simulink model "with_demand_res_final_v5"  (R2024a)
settings: Solver=VariableStepAuto  StartTime=0.0  StopTime=24  RelTol=1e-3
InitFcn:
  | set_param(bdroot, 'StopTime', num2str(stop_time));
values from neighbouring files (symbols this model uses):
  fnom = 50    [initial_conditions.m]
  L_H_20kv = X_20kv_ohm/(2*pi*fnom)    (= 0.00126369024815)    [initial_conditions.m]
  L_H_400v = X_400v_ohm/(2*pi*fnom)    (= 0.00022600001919)    [initial_conditions.m]
  Pload_opt_nngwo_comb_cost = Pload_opt_nn    [gwo_nn_comb_cost.m]
  R_20kv = 0.576    [initial_conditions.m]
  R_400v = 0.410    (= 0.41)    [initial_conditions.m]
  Vph_ph_rms_nom_supply = 20e3    (= 20000)    [initial_conditions.m]
undefined symbols (not defined in the file or in its folder): D1, Delta
libraries: spsRMSLib x14, spsThreePhaseVIMeasurementLib x8, spsPowerPositiveSequenceLib x7, spsPLL3phLib x6, spsStairGeneratorLib x4, spsSeriesRLCBranchLib x3, spsThreePhasePISectionLineLib x2, spsThreePhaseTransformerTwoWindingsLib x2, spsThreePhaseSeriesRLCBranchLib x2, spsThreePhaseSeriesRLCLoadLib x2, slpidlib x2, spsabctodq0Lib x2
(part 1 of 2)
settings Model: Creator=arisi  LastModifiedBy=arisi
settings DataIOCC: ReturnWorkspaceOutputsName=with_demand_res

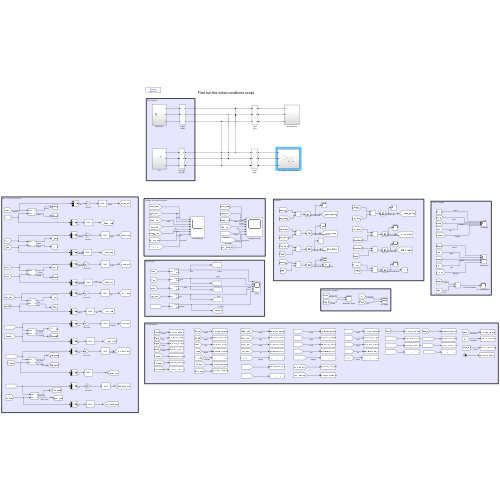
[thumbnail: Simulink's stored preview of the top-level diagram]
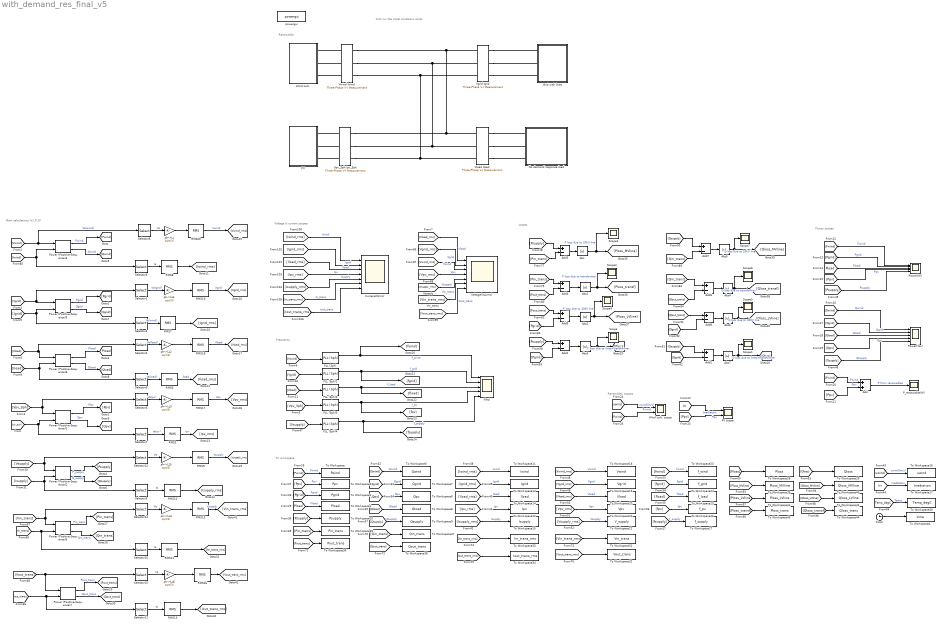
== system with_demand_res_final_v5 ==
  note: Voltage & current scopes
  note: First run the initial conditions script
  note: Losses
  note: Main calculations (V,I,P,Q)
  note: Frequency
  note: To workspace
  note: Renewable
  note: Renewbles' scopes
  note: Power scopes
  Abs{,1..7} (8 alike) : Abs  SaturateOnIntegerOverflow=off
  Add : Sum
  Add{1..8} (8 alike) : Sum  Inputs=+-
  Clock : Clock
  Currenet(Irms) : Scope  NumInputPorts=7
  Grid with lines : Subsystem
  No demand response load : Subsystem
  PLL (3ph){,1..4} (5 alike) : spsPLL3phLib/PLL (3ph)  Fmin=45  Par_Init=[0, 50]  ParK=[180, 3200, 1]  TcD=1e-4  MaxRateChangeFreq=12  FilterCutOffFreq=25  Ts=0  AGC=on
  PV : Subsystem
  PV scope : Scope  NumInputPorts=2
  P_renewable(W) : Scope
  Power (Positive-Sequence){1..7} (7 alike) : spsPowerPositiveSequenceLib/Power (Positive-Sequence)  Freq=50  Vinit=[0, 0]  Iinit=[0, 0]  Ts=0
      settings: LibrarySourceBlock=|
      | sps_lib/Sensors and Measurements/Power
      | (Positive-Sequence)
  Power(Var) : Scope  NumInputPorts=5
  Power(W) : Scope  NumInputPorts=5
  RMS{2,6..8,10..11,13} (7 alike) : spsRMSLib/RMS  TrueRMS=on  Freq=50  RMSInit=0  Ts=0
  RMS15 : spsRMSLib/RMS  TrueRMS=on  Freq=50  RMSInit=20e3  Ts=0
  RMS{16..20} (5 alike) : spsRMSLib/RMS  TrueRMS=on  Freq=50  RMSInit=400  Ts=0
  RMS9 : spsRMSLib/RMS  TrueRMS=on  Freq=50  RMSInit=20e3  Ts=0
  Scope{,1..7} (8 alike) : Scope
  Selector{1..12,14..15} (14 alike) : Selector  InputPortWidth=3  IndexOptions=Index vector (dialog)  Indices=1  OutputSizes=1
  To Workspace : ToWorkspace  VariableName=Pwind  SampleTime=-1
      settings: Save2DSignal=2-D array (concatenate along first dimension)
  To Workspace1 : ToWorkspace  VariableName=Pload  SampleTime=-1
      settings: Save2DSignal=2-D array (concatenate along first dimension)
  To Workspace10 : ToWorkspace  VariableName=Psupply  SampleTime=-1
      settings: Save2DSignal=2-D array (concatenate along first dimension)
  To Workspace11 : ToWorkspace  VariableName=Iwind  SampleTime=-1
      settings: Save2DSignal=2-D array (concatenate along first dimension)
  To Workspace12 : ToWorkspace  VariableName=Ipv  SampleTime=-1
      settings: Save2DSignal=2-D array (concatenate along first dimension)
  To Workspace13 : ToWorkspace  VariableName=Igrid  SampleTime=-1
      settings: Save2DSignal=2-D array (concatenate along first dimension)
  To Workspace14 : ToWorkspace  VariableName=Iload  SampleTime=-1
      settings: Save2DSignal=2-D array (concatenate along first dimension)
  To Workspace15 : ToWorkspace  VariableName=Isupply  SampleTime=-1
      settings: Save2DSignal=2-D array (concatenate along first dimension)
  To Workspace16 : ToWorkspace  VariableName=uwind  SampleTime=-1
      settings: Save2DSignal=2-D array (concatenate along first dimension)
  To Workspace17 : ToWorkspace  VariableName=Irradiation  SampleTime=-1
      settings: Save2DSignal=2-D array (concatenate along first dimension)
  To Workspace18 : ToWorkspace  VariableName=Vwind  SampleTime=-1
      settings: Save2DSignal=2-D array (concatenate along first dimension)
  To Workspace19 : ToWorkspace  VariableName=Vgrid  SampleTime=-1
      settings: Save2DSignal=2-D array (concatenate along first dimension)
  To Workspace2 : ToWorkspace  VariableName=Pgrid  SampleTime=-1
      settings: Save2DSignal=2-D array (concatenate along first dimension)
  To Workspace20 : ToWorkspace  VariableName=Vload  SampleTime=-1
      settings: Save2DSignal=2-D array (concatenate along first dimension)
  To Workspace21 : ToWorkspace  VariableName=Vpv  SampleTime=-1
      settings: Save2DSignal=2-D array (concatenate along first dimension)
  To Workspace22 : ToWorkspace  VariableName=V_supply  SampleTime=-1
      settings: Save2DSignal=2-D array (concatenate along first dimension)
  To Workspace23 : ToWorkspace  VariableName=f_wind  SampleTime=-1
      settings: Save2DSignal=2-D array (concatenate along first dimension)
  To Workspace24 : ToWorkspace  VariableName=f_grid  SampleTime=-1
      settings: Save2DSignal=2-D array (concatenate along first dimension)
  To Workspace25 : ToWorkspace  VariableName=f_load  SampleTime=-1
      settings: Save2DSignal=2-D array (concatenate along first dimension)
  To Workspace26 : ToWorkspace  VariableName=f_pv  SampleTime=-1
      settings: Save2DSignal=2-D array (concatenate along first dimension)
  To Workspace27 : ToWorkspace  VariableName=f_supply  SampleTime=-1
      settings: Save2DSignal=2-D array (concatenate along first dimension)
  To Workspace28 : ToWorkspace  VariableName=Ploss  SampleTime=-1
      settings: Save2DSignal=2-D array (concatenate along first dimension)
  To Workspace29 : ToWorkspace  VariableName=Qloss  SampleTime=-1
      settings: Save2DSignal=2-D array (concatenate along first dimension)
  To Workspace3 : ToWorkspace  VariableName=Ppv  SampleTime=-1
      settings: Save2DSignal=2-D array (concatenate along first dimension)
  To Workspace30 : ToWorkspace  VariableName=Temp_degC  SampleTime=-1
      settings: Save2DSignal=2-D array (concatenate along first dimension)
  To Workspace31 : ToWorkspace  VariableName=Vin_trans  SampleTime=-1
      settings: Save2DSignal=2-D array (concatenate along first dimension)
  To Workspace32 : ToWorkspace  VariableName=Vout_trans  SampleTime=-1
      settings: Save2DSignal=2-D array (concatenate along first dimension)
  To Workspace33 : ToWorkspace  VariableName=Iin_trans_rms  SampleTime=-1
      settings: Save2DSignal=2-D array (concatenate along first dimension)
  To Workspace34 : ToWorkspace  VariableName=Iout_trans_rms  SampleTime=-1
      settings: Save2DSignal=2-D array (concatenate along first dimension)
  To Workspace35 : ToWorkspace  VariableName=Pin_trans  SampleTime=-1
      settings: Save2DSignal=2-D array (concatenate along first dimension)
  To Workspace36 : ToWorkspace  VariableName=Pout_trans  SampleTime=-1
      settings: Save2DSignal=2-D array (concatenate along first dimension)
  To Workspace37 : ToWorkspace  VariableName=Qin_trans  SampleTime=-1
      settings: Save2DSignal=2-D array (concatenate along first dimension)
  To Workspace38 : ToWorkspace  VariableName=Qout_trans  SampleTime=-1
      settings: Save2DSignal=2-D array (concatenate along first dimension)
  To Workspace39 : ToWorkspace  VariableName=Ploss_MVline  SampleTime=-1
      settings: Save2DSignal=2-D array (concatenate along first dimension)
  To Workspace4 : ToWorkspace  VariableName=time  SampleTime=-1
      settings: Save2DSignal=2-D array (concatenate along first dimension)
  To Workspace40 : ToWorkspace  VariableName=Qloss_MVline  SampleTime=-1
      settings: Save2DSignal=2-D array (concatenate along first dimension)
  To Workspace41 : ToWorkspace  VariableName=Ploss_LVline  SampleTime=-1
      settings: Save2DSignal=2-D array (concatenate along first dimension)
  To Workspace42 : ToWorkspace  VariableName=Qloss_LVline  SampleTime=-1
      settings: Save2DSignal=2-D array (concatenate along first dimension)
  To Workspace43 : ToWorkspace  VariableName=Ploss_trans  SampleTime=-1
      settings: Save2DSignal=2-D array (concatenate along first dimension)
  To Workspace44 : ToWorkspace  VariableName=Qloss_trans  SampleTime=-1
      settings: Save2DSignal=2-D array (concatenate along first dimension)
  To Workspace5 : ToWorkspace  VariableName=Qwind  SampleTime=-1
      settings: Save2DSignal=2-D array (concatenate along first dimension)
  To Workspace6 : ToWorkspace  VariableName=Qpv  SampleTime=-1
      settings: Save2DSignal=2-D array (concatenate along first dimension)
  To Workspace7 : ToWorkspace  VariableName=Qgrid  SampleTime=-1
      settings: Save2DSignal=2-D array (concatenate along first dimension)
  To Workspace8 : ToWorkspace  VariableName=Qload  SampleTime=-1
      settings: Save2DSignal=2-D array (concatenate along first dimension)
  To Workspace9 : ToWorkspace  VariableName=Qsupply  SampleTime=-1
      settings: Save2DSignal=2-D array (concatenate along first dimension)
  Vgrid Igrid : spsThreePhaseVIMeasurementLib/Three-Phase V-I Measurement  VoltageMeasurement=phase-to-ground  SetLabelV=on  LabelV=Vgrid  Vpu=off  VpuLL=off  CurrentMeasurement=yes  SetLabelI=on  LabelI=Igrid  Ipu=off  Pbase=100e6  Vbase=500e3  OutputType=Complex  PhasorSimulation=off  PSBequivalent=0
  Vload Iload : spsThreePhaseVIMeasurementLib/Three-Phase V-I Measurement  VoltageMeasurement=phase-to-ground  SetLabelV=on  LabelV=Vload  Vpu=off  VpuLL=off  CurrentMeasurement=yes  SetLabelI=on  LabelI=Iload  Ipu=off  Pbase=100e6  Vbase=500e3  OutputType=Complex  PhasorSimulation=off  PSBequivalent=0
  Voltage(VLLrms) : Scope  NumInputPorts=7
  Vpv_3ph Ipv_3ph : spsThreePhaseVIMeasurementLib/Three-Phase V-I Measurement  VoltageMeasurement=phase-to-ground  SetLabelV=on  LabelV=Vpv_3ph  Vpu=off  VpuLL=off  CurrentMeasurement=yes  SetLabelI=on  LabelI=Ipv_3ph  Ipu=off  Pbase=100e6  Vbase=500e3  OutputType=Complex  PhasorSimulation=off  PSBequivalent=0
  Vwind Iwind : spsThreePhaseVIMeasurementLib/Three-Phase V-I Measurement  VoltageMeasurement=phase-to-ground  SetLabelV=on  LabelV=Vwind  Vpu=off  VpuLL=off  CurrentMeasurement=yes  SetLabelI=on  LabelI=Iwind  Ipu=off  Pbase=100e6  Vbase=500e3  OutputType=Complex  PhasorSimulation=off  PSBequivalent=0
  Wind turb. : Subsystem
  Wind turb. scope : Scope  NumInputPorts=2
  f(Hz) : Scope  NumInputPorts=5
  ph->LL{,1..6} (7 alike) : Gain  Gain=sqrt(3)
  powergui : spspowerguiLib/powergui  Priority=1  SimulationMode=Discrete  SampleTime=6.06e-6  frequency=60  Iterations=50  frequencyindice=50  Pbase=100e6  ErrMax=1e-4  UnitsV=kV  UnitsW=MW  buscounter=0  FunctionMessages=off  echomessages=off  EnableUseOfTLC=off  CurrentSourceSwitches=off  DisableSnubberDevices=off  DisableRonSwitches=off  DisableVfSwitches=off  DisplayEquations=off  AutomaticDiscreteSolvers=off  SolverType=Tustin  Interpol=off  ExternalGateDelay=off  methode=off  Ts=0  x0status=blocks  SPID=off  SwTol=0  HookPort=off  NonlinearTolerance=1e-4  nMaxIteration=15  ContinueOnMaxIteration=off  RestoreLinks=warning  ResistiveCurrentMeasurement=off  Frange=[0:2:500]  Ylog=off  Xlog=on  ShowGrid=off  save=off  variable=ZData  structure=VaIa_Grid  ZoomFFT=off  StartTime=1.4  cycles=3  DisplayStyle=1  fundamental=60  FreqAxis=on  MaxFrequency=5000  frequencyindicesteady=1  RmsSteady=1  display=off
  tag scope: Pload=global
  wires:
  Power (Positive-Sequence)5/2 -> [Qgrid]  "Qgrid"
  Selector6/1 -> ph->LL3/1  "Va(pv)"
  PLL (3ph)1/1 -> f(Hz)/2, [fgrid]  "f_grid"
  Power (Positive-Sequence)4/2 -> [Qwind]  "Qwind"
  [Irr] -> PV scope/1  "Irradiation"
  [Qpv] -> Power(Var)/4  "Qpv"
  [Ppv] -> PV scope/2  "Ppv"
  [Pwind] -> Wind turb. scope/2  "Pwind"
  Power (Positive-Sequence)1/2 -> [Qpv]  "Qpv"
  [Vpv_3ph] -> Power (Positive-Sequence)1/1, Selector6/1
  [Vload] -> Selector2/1, Power (Positive-Sequence)6/1
  [Ppv] -> Add/2  "Ppv"
  [uwind] -> Wind turb. scope/1  "uwind(m/s)"
  [Pload] -> Power(W)/3  "Pload"
  RMS7/1 -> [Igrid_rms]
  Selector2/1 -> ph->LL2/1  "Va(load)"
  ph->LL3/1 -> RMS17/1
  RMS6/1 -> [Iload_rms]  "Iload"
  Power (Positive-Sequence)6/2 -> [Qload]  "Qload"
  Power (Positive-Sequence)1/1 -> [Ppv]  "Plpv"
  Add/1 -> P_renewable(W)/1  "P from renewables"
  [Pwind] -> Add/1  "Pwind"
  [Qgrid] -> Power(Var)/2  "Qgrid"
  [Qwind] -> Power(Var)/1  "Qwind"
  [Qload] -> Power(Var)/3  "Qload"
  [Pgrid] -> Power(W)/2  "Pgrid"
  PLL (3ph)2/1 -> f(Hz)/3, [fload]  "f_load"
  Power (Positive-Sequence)5/1 -> [Pgrid]  "Pgrid"
  Selector1/1 -> ph->LL1/1  "Va(grid)"
  [Vgrid] -> Selector1/1, Power (Positive-Sequence)5/1
  RMS8/1 -> [Iwind_rms]
  [Vpv_3ph] -> PLL (3ph)3/1
  RMS2/1 -> [Ipv_rms]  "Ipv"
  [Pwind] -> Power(W)/1  "Pwind"
  [Vload] -> PLL (3ph)2/1
  Power (Positive-Sequence)4/1 -> [Pwind]  "Pwind"
  ph->LL1/1 -> RMS19/1
  PLL (3ph)3/1 -> [fpv], f(Hz)/4  "f_pv"
  ph->LL2/1 -> RMS18/1
  Selector5/1 -> RMS8/1  "Ia"
  [Ppv] -> Power(W)/4  "Ppv"
  Selector4/1 -> RMS7/1  "Ia(wind)"
  Selector3/1 -> RMS6/1  "Ia(load)"
  PLL (3ph)/1 -> f(Hz)/1, [fwind]  "f_wind"
  Selector7/1 -> RMS2/1  "Ia(pv)"
  [Vwind] -> Selector8/1, Power (Positive-Sequence)4/1  "Va(wind)"
  Power (Positive-Sequence)6/1 -> [Pload]  "Pload"
  [Vgrid] -> PLL (3ph)1/1
  [Vwind] -> PLL (3ph)/1
  [Pwind] -> To Workspace/1  "Pwind"
  [Ppv] -> To Workspace3/1  "Ppv"
  [Pgrid] -> To Workspace2/1  "Pgrid"
  [Pload] -> To Workspace1/1  "Pload"
  Clock/1 -> To Workspace4/1
  ph->LL5/1 -> RMS9/1
  Power (Positive-Sequence)2/1 -> [Psupply]  "P_supply"
  Selector12/1 -> ph->LL5/1  "Va"
  Power (Positive-Sequence)2/2 -> [Qsupply]  "Q_supply"
  [Vsupply] -> Selector12/1, Power (Positive-Sequence)2/1
  Selector9/1 -> RMS10/1  "Ia"
  RMS10/1 -> [Isupply_rms]
  [Qwind] -> To Workspace5/1  "Qwind"
  [Qgrid] -> To Workspace7/1  "Qgrid"
  [Qpv] -> To Workspace6/1  "Qpv"
  [Qload] -> To Workspace8/1  "Qload"
  [Qsupply] -> To Workspace9/1  "Qsupply"
  [Psupply] -> To Workspace10/1
  [Iwind_rms] -> To Workspace11/1  "Iwind"
  [Igrid_rms] -> To Workspace13/1  "Igrid"
  [Iload_rms] -> To Workspace14/1  "Iload"
  [Ipv_rms] -> To Workspace12/1  "Ipv"
  [Isupply_rms] -> To Workspace15/1  "Isupply"
  [uwind] -> To Workspace16/1  "uwind(m/s)"
  [Irr] -> To Workspace17/1  "Irradiation"
  [Psupply] -> Power(W)/5  "Psupply"
  [Qsupply] -> Power(Var)/5  "Qsupply"
  [Vsupply] -> PLL (3ph)4/1
  PLL (3ph)4/1 -> f(Hz)/5, [fsupply]  "f_supply"
  [Vwind_rms] -> To Workspace18/1  "Vwind"
  [Vgrid_rms] -> To Workspace19/1  "Vgrid"
  [Vload_rms] -> To Workspace20/1  "Vload"
  [Vpv_rms] -> To Workspace21/1  "Vpv"
  [Vsupply_rms] -> To Workspace22/1  "Vsupply"
  [fwind] -> To Workspace23/1  "fwind"
  [fgrid] -> To Workspace24/1  "fgrid"
  [fload] -> To Workspace25/1  "fload"
  [fpv] -> To Workspace26/1  "fpv"
  [fsupply] -> To Workspace27/1  "f_supply"
  [Psupply] -> Add1/1
  [Pgrid] -> Add1/2
  [Qsupply] -> Add2/1
  [Qgrid] -> Add2/2
  [Ploss] -> To Workspace28/1
  [Qloss] -> To Workspace29/1
  [Temp_degC] -> To Workspace30/1  "Temp"
  Selector11/1 -> RMS13/1  "Ia"
  Selector10/1 -> RMS11/1  "Ia"
  [Vout_trans] -> Power (Positive-Sequence)7/1, Selector15/1
  Power (Positive-Sequence)3/1 -> [Pin_trans]  "Pin_trans"
  Power (Positive-Sequence)3/2 -> [Qin_trans]  "Qin_trans"
  Power (Positive-Sequence)7/2 -> [Qout_trans]  "Qout_trans"
  Power (Positive-Sequence)7/1 -> [Pout_trans]  "Pout_trans"
  RMS11/1 -> [Iin_trans_rms]
  [Vin_trans_rms] -> To Workspace31/1
  RMS13/1 -> [Iout_trans_rms]
  [Iin_trans_rms] -> To Workspace33/1
  [Iout_trans_rms] -> To Workspace34/1
  [Vout_trans_rms] -> To Workspace32/1
  [Pin_trans] -> To Workspace35/1
  [Pout_trans] -> To Workspace36/1
  [Qin_trans] -> To Workspace37/1
  [Qout_trans] -> To Workspace38/1
  [Pin_trans] -> Add3/2
  [Psupply] -> Add3/1
  [Pin_trans] -> Add4/1
  [Pout_trans] -> Add4/2
  [Pout_trans] -> Add5/1
  [Pgrid] -> Add5/2
  [Qin_trans] -> Add6/1
  [Qout_trans] -> Add6/2
  [Qin_trans] -> Add7/2
  [Qsupply] -> Add7/1
  [Qgrid] -> Add8/2
  [Qout_trans] -> Add8/1
  [Ploss_MVline] -> To Workspace39/1
  [Qloss_MVline] -> To Workspace40/1
  [Qloss_LVline] -> To Workspace42/1
  [Ploss_LVline] -> To Workspace41/1
  [Qloss_transf] -> To Workspace44/1
  [Ploss_transf] -> To Workspace43/1
  [Iwind] -> Selector5/1, Power (Positive-Sequence)4/2
  [Igrid] -> Selector4/1, Power (Positive-Sequence)5/2
  [Iload] -> Selector3/1, Power (Positive-Sequence)6/2
  [Ipv_3ph] -> Selector7/1, Power (Positive-Sequence)1/2
  [Isupply] -> Selector9/1, Power (Positive-Sequence)2/2
  [Vin_trans] -> Selector14/1, Power (Positive-Sequence)3/1
  [Iin_trans] -> Selector10/1, Power (Positive-Sequence)3/2
  [Iout_trans] -> Selector11/1, Power (Positive-Sequence)7/2
  Selector14/1 -> ph->LL4/1  "Va"
  ph->LL4/1 -> RMS15/1
  Selector15/1 -> ph->LL6/1  "Va"
  ph->LL6/1 -> RMS16/1
  RMS19/1 -> [Vgrid_rms]  "Vgrid"
  RMS18/1 -> [Vload_rms]  "Vload"
  RMS17/1 -> [Vpv_rms]  "Vpv"
  RMS9/1 -> [Vsupply_rms]  "Vsupply"
  RMS15/1 -> [Vin_trans_rms]  "Vsupply"
  RMS16/1 -> [Vout_trans_rms]
  [Vload_rms] -> Voltage(VLLrms)/1  "Vload"
  [Vgrid_rms] -> Voltage(VLLrms)/2  "Vgrid"
  [Vwind_rms] -> Voltage(VLLrms)/3  "Vwind"
  [Vpv_rms] -> Voltage(VLLrms)/4  "Vpv"
  [Vsupply_rms] -> Voltage(VLLrms)/5  "Vsupply"
  [Vin_trans_rms] -> Voltage(VLLrms)/6  "Vin_trans"
  [Vout_trans_rms] -> Voltage(VLLrms)/7  "Vout_trans"
  [Iwind_rms] -> Currenet(Irms)/1  "Iwind"
  [Igrid_rms] -> Currenet(Irms)/2  "Igird"
  [Iload_rms] -> Currenet(Irms)/3  "Iload"
  [Ipv_rms] -> Currenet(Irms)/4  "Ipv"
  [Isupply_rms] -> Currenet(Irms)/5  "Isupply"
  [Iin_trans_rms] -> Currenet(Irms)/6  "In_trans"
  [Iout_trans_rms] -> Currenet(Irms)/7  "Iout_trans"
  Add3/1 -> Abs/1
  Abs/1 -> Scope2/1, [Ploss_MVline]  "P loss due to 20kV line"
  Add4/1 -> Abs1/1
  Abs1/1 -> Scope3/1, [Ploss_transf]  "P loss due to transformer"
  Add5/1 -> Abs2/1
  Abs2/1 -> Scope4/1, [Ploss_LVline]  "P loss due to 400V line"
  Add1/1 -> Abs3/1
  Abs3/1 -> Scope/1, [Ploss]  "P loss due to lines+transformer"
  Add2/1 -> Abs7/1
  Abs7/1 -> [Qloss], Scope1/1  "Q loss due to lines+transformer"
  Add8/1 -> Abs6/1
  Abs6/1 -> [Qloss_LVline], Scope5/1  "Q loss due to 400V line"
  Add6/1 -> Abs4/1
  Abs4/1 -> [Qloss_transf], Scope6/1  "Q loss due to transformer"
  Add7/1 -> Abs5/1
  Abs5/1 -> [Qloss_MVline], Scope7/1  "Q loss due to 20kV line"
  ph->LL/1 -> RMS20/1
  Selector8/1 -> ph->LL/1  "Va"
  RMS20/1 -> [Vwind_rms]  "Vwind"
  connections:
  Vload Iload/LConn2 -- Vpv_3ph Ipv_3ph/RConn2 -- Vwind Iwind/RConn2 -- Vgrid Igrid/RConn2
  Vload Iload/LConn3 -- Vpv_3ph Ipv_3ph/RConn3 -- Vwind Iwind/RConn3 -- Vgrid Igrid/RConn3
  Vload Iload/LConn1 -- Vwind Iwind/RConn1 -- Vgrid Igrid/RConn1 -- Vpv_3ph Ipv_3ph/RConn1
  Vload Iload/RConn1 -- No demand response load/LConn1
  Vload Iload/RConn2 -- No demand response load/LConn2
  Vload Iload/RConn3 -- No demand response load/LConn3
  Vwind Iwind/LConn2 -- Wind turb./LConn2
  Vpv_3ph Ipv_3ph/LConn3 -- PV/RConn3
  Vwind Iwind/LConn3 -- Wind turb./LConn3
  Vwind Iwind/LConn1 -- Wind turb./LConn1
  Vpv_3ph Ipv_3ph/LConn2 -- PV/RConn2
  Vpv_3ph Ipv_3ph/LConn1 -- PV/RConn1
  Vgrid Igrid/LConn3 -- Grid with lines/RConn3
  Vgrid Igrid/LConn1 -- Grid with lines/RConn1
  Vgrid Igrid/LConn2 -- Grid with lines/RConn2

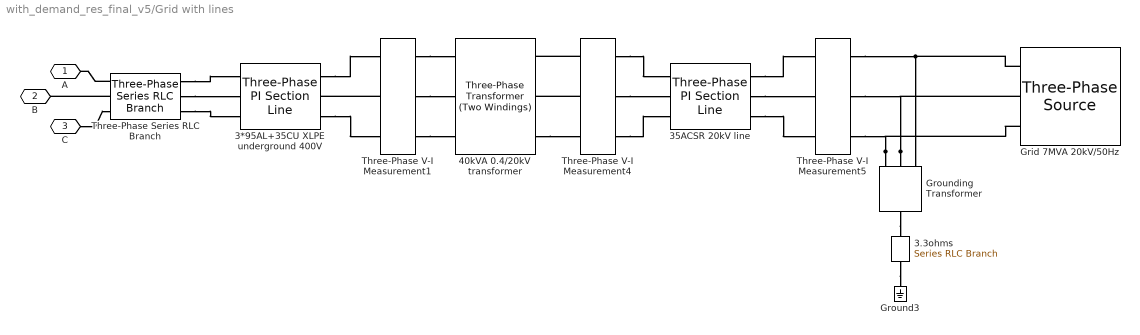
== system with_demand_res_final_v5/Grid with lines ==
  3*95AL+35CU XLPE underground 400V : spsThreePhasePISectionLineLib/Three-Phase PI Section Line  LConnTagsString=a|b|c  RConnTagsString=A|B|C  Length=km_400v  Frequency=fnom  Resistances=[ R_400v 0.724]  Inductances="[ L_H_400v  1.595/(2*pi*50)]"  Capacitances=[60e-9 7.751e-9]
  "3.3ohms " : spsSeriesRLCBranchLib/Series RLC Branch  LConnTagsString=__new0  RConnTagsString=__new0  BranchType=R  Resistance=3.3  Inductance=[]  SetiL0=off  InitialCurrent=0  Capacitance=[]  Setx0=off  InitialVoltage=0  Measurements=None
  35ACSR 20kV line : spsThreePhasePISectionLineLib/Three-Phase PI Section Line  LConnTagsString=a|b|c  RConnTagsString=A|B|C  Length=km_20kv  Frequency=fnom  Resistances=[ R_20kv 0.724]  Inductances="[ L_H_20kv  1.595/(2*pi*50)]"  Capacitances=[50e-9 7.751e-9]
  40kVA 0.4/20kV transformer : spsThreePhaseTransformerTwoWindingsLib/Three-Phase Transformer (Two Windings)  Winding1Connection=Yg  Winding2Connection=Delta (D1)  CoreType=Three single-phase transformers  SetSaturation=off  Hysteresis=off  DataFile='hysteresis'  SetInitialFlux=off  Measurements=None  UNITS=pu  NominalPower=nominal_trans_param  Winding1=winding_1_param  Winding2=winding_2_param  Rm=Lm_pu  Lm=Rm_pu  L0=0.5  Saturation=[ 0,0 ; 0.0024,1.2 ; 1.0,1.52 ]  InitialFluxes=[ 0.8 , -0.8 , 0.7 ]  BreakLoop=off  DiscreteSolver=Trapezoidal iterative  DataType=off  TransfoNumber=1
  "Grid 7MVA 20kV/50Hz " : spsThreePhaseSourceLib/Three-Phase Source  InternalConnection=Yg  VoltagePhases=off  Voltage=Vph_ph_rms_nom_supply  PhaseAngle=0  Voltage_phases=[25e3 25e3 25e3]/sqrt(3)  PhaseAngles_phases=[0 -120 +120]  Frequency=fnom  NonIdealSource=on  SpecifyImpedance=on  Resistance=0.8929  Inductance=16.58e-3  ShortCircuitLevel=Ssupply  BaseVoltage=Vph_ph_rms_nom_supply  XRratio=XRratio  BusType=swing  Pref=0  Qref=0  Prefabc=[10e3, 10e3, 10e3]  Qrefabc=[0, 0, 0]  Qmin=-inf  Qmax=inf
  Ground3 : spsGroundLib/Ground  LConnTagsString=a
  "Grounding Transformer " : spsGroundingTransformerLib/Grounding Transformer   UNITS=pu  NominalPower="[100e6   50]"  NominalVoltage=20e3  ZeroSequenceImpedance_pu=[0.025 0.75]  MagnetizationBranch_pu=[500 500]  ZeroSequenceImpedance_SI=[0.052083 589.05]  MagnetizationBranch_SI=[1041.7 3.927e+005]  Measurements=None
      settings: LibrarySourceBlock=|
      | sps_lib/Power Grid Elements/Grounding
      | Transformer
  Three-Phase Series RLC Branch : spsThreePhaseSeriesRLCBranchLib/Three-Phase Series RLC Branch  LConnTagsString=A|B|C  RConnTagsString=A|B|C  BranchType=R  Resistance=1e-3  Inductance=1e-3  Capacitance=1e-6  Measurements=None
  Three-Phase V-I Measurement1 : spsThreePhaseVIMeasurementLib/Three-Phase V-I Measurement  VoltageMeasurement=phase-to-ground  SetLabelV=on  LabelV=Vout_trans  Vpu=off  VpuLL=off  CurrentMeasurement=yes  SetLabelI=on  LabelI=Iout_trans  Ipu=off  Pbase=100e6  Vbase=500e3  OutputType=Complex  PhasorSimulation=off  PSBequivalent=0
  Three-Phase V-I Measurement4 : spsThreePhaseVIMeasurementLib/Three-Phase V-I Measurement  VoltageMeasurement=phase-to-ground  SetLabelV=on  LabelV=Vin_trans  Vpu=off  VpuLL=off  CurrentMeasurement=yes  SetLabelI=on  LabelI=Iin_trans  Ipu=off  Pbase=100e6  Vbase=500e3  OutputType=Complex  PhasorSimulation=off  PSBequivalent=0
  Three-Phase V-I Measurement5 : spsThreePhaseVIMeasurementLib/Three-Phase V-I Measurement  VoltageMeasurement=phase-to-ground  SetLabelV=on  LabelV=Vsupply  Vpu=off  VpuLL=off  CurrentMeasurement=yes  SetLabelI=on  LabelI=Isupply  Ipu=off  Pbase=100e6  Vbase=500e3  OutputType=Complex  PhasorSimulation=off  PSBequivalent=0
  A : PMIOPort  Side=Right
  B : PMIOPort  Port=2  Side=Right
  C : PMIOPort  Port=3  Side=Right
  connections:
  Three-Phase Series RLC Branch/RConn1 -- A/RConn1
  Three-Phase Series RLC Branch/LConn1 -- 3*95AL+35CU XLPE underground 400V/RConn1
  3*95AL+35CU XLPE underground 400V/LConn1 -- Three-Phase V-I Measurement1/RConn1
  "Grounding Transformer "/LConn2 -- "Grid 7MVA 20kV/50Hz "/RConn2 -- Three-Phase V-I Measurement5/LConn2
  "Grid 7MVA 20kV/50Hz "/RConn1 -- "Grounding Transformer "/LConn1 -- Three-Phase V-I Measurement5/LConn1
  Three-Phase V-I Measurement1/RConn2 -- 3*95AL+35CU XLPE underground 400V/LConn2
  Three-Phase V-I Measurement4/RConn1 -- 40kVA 0.4/20kV transformer/LConn1
  "Grounding Transformer "/RConn1 -- "3.3ohms "/LConn1
  35ACSR 20kV line/LConn3 -- Three-Phase V-I Measurement5/RConn3
  Three-Phase V-I Measurement1/LConn2 -- 40kVA 0.4/20kV transformer/RConn2
  Three-Phase V-I Measurement1/LConn1 -- 40kVA 0.4/20kV transformer/RConn1
  Three-Phase Series RLC Branch/LConn2 -- 3*95AL+35CU XLPE underground 400V/RConn2
  Three-Phase V-I Measurement4/LConn1 -- 35ACSR 20kV line/RConn1
  Three-Phase Series RLC Branch/LConn3 -- 3*95AL+35CU XLPE underground 400V/RConn3
  "Grounding Transformer "/LConn3 -- "Grid 7MVA 20kV/50Hz "/RConn3 -- Three-Phase V-I Measurement5/LConn3
  35ACSR 20kV line/LConn2 -- Three-Phase V-I Measurement5/RConn2
  35ACSR 20kV line/LConn1 -- Three-Phase V-I Measurement5/RConn1
  "3.3ohms "/RConn1 -- Ground3/LConn1
  Three-Phase V-I Measurement4/RConn2 -- 40kVA 0.4/20kV transformer/LConn2
  Three-Phase V-I Measurement4/LConn3 -- 35ACSR 20kV line/RConn3
  Three-Phase V-I Measurement4/LConn2 -- 35ACSR 20kV line/RConn2
  40kVA 0.4/20kV transformer/LConn3 -- Three-Phase V-I Measurement4/RConn3
  Three-Phase V-I Measurement1/LConn3 -- 40kVA 0.4/20kV transformer/RConn3
  Three-Phase Series RLC Branch/RConn2 -- B/RConn1
  3*95AL+35CU XLPE underground 400V/LConn3 -- Three-Phase V-I Measurement1/RConn3
  C/RConn1 -- Three-Phase Series RLC Branch/RConn3

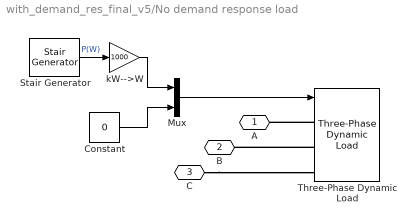
== system with_demand_res_final_v5/No demand response load ==
  Constant : Constant  Value=0
  Mux : Mux  Inputs=2
  Stair Generator : spsStairGeneratorLib/Stair Generator  t=no_drload_time  e=(Pload_opt_nngwo_comb_cost)'  Ts=0
  Three-Phase Dynamic Load : spsThreePhaseDynamicLoadLib/Three-Phase Dynamic Load  NominalVoltage=[ 400 50 ]  ActiveReactivePowers=[6e3 0]  PositiveSequence=[0.994 -11.8]  ExternalControl=on  NpNq=[1.3 2]  TimeConstants="[0  0  0  0]"  MinimumVoltage=0.7  Tfilter=1e-4  LoadFlowParameters=[4,0,0,0,0]
      settings: LibrarySourceBlock=|
      | sps_lib/Passives/Three-Phase
      | Dynamic Load
  kW-->W : Gain  Gain=1000
  A : PMIOPort  Side=Left
  B : PMIOPort  Port=2  Side=Left
  C : PMIOPort  Port=3  Side=Left
  wires:
  Mux/1 -> Three-Phase Dynamic Load/1
  Stair Generator/1 -> kW-->W/1  "P(W)"
  Constant/1 -> Mux/2
  kW-->W/1 -> Mux/1
  connections:
  C/RConn1 -- Three-Phase Dynamic Load/LConn3
  Three-Phase Dynamic Load/LConn1 -- A/RConn1
  Three-Phase Dynamic Load/LConn2 -- B/RConn1

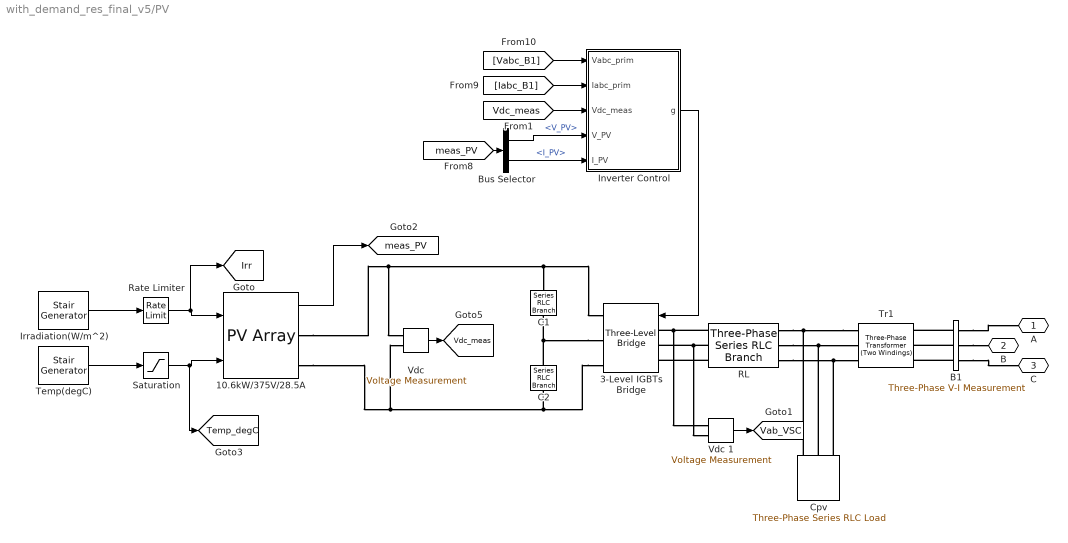
== system with_demand_res_final_v5/PV ==
  10.6kW/375V/28.5A : spsPVArrayLib/PV Array  Npar=4  Nser=13  PlotType=array @ 25 deg.C & specified irradiances  S_vec="[ 1000  500  100 ]"  Temp_C_vec="[ 45 25  ]"  ModuleName=Solartech Power SPM205P  PlotWhenSelected=off  Pm=205.056  Ncell=60  Voc=37.1  Isc=8.07  Vm=28.8  Im=7.12  beta_Voc_pc=-0.36403  alpha_Isc_pc=0.051128  beta_Voc=-0.13506  alpha_Isc=0.004126  IL=8.1521  I0=3.0369e-10  nI=1.006  Rsh=52.6281  Rs=0.53549  RobustModel=off  RobustCellTemperature=313.3991  BAL=on  Tc=1e-6  Tfilter=5e-5
  3-Level IGBTs Bridge : spsThreeLevelBridgeLib/Three-Level Bridge  Arms=3  SnubberResistance=1e6  SbubberCapacitance=inf  Device=IGBT / Diodes  Ron=1e-3  ForwardVoltages="[  0  0 ]"  Measurements=None
      settings: AttributesFormatString=\n  LibrarySourceBlock=sps_lib/Power Electronics/Three-Level Bridge
  B1 : spsThreePhaseVIMeasurementLib/Three-Phase V-I Measurement  VoltageMeasurement=phase-to-ground  SetLabelV=on  LabelV=Vabc_B1  Vpu=off  VpuLL=off  CurrentMeasurement=yes  SetLabelI=on  LabelI=Iabc_B1  Ipu=off  Pbase=100e6  Vbase=500e3  OutputType=Magnitude  PhasorSimulation=off  PSBequivalent=0
  Bus Selector : BusSelector  OutputSignals=V_PV,I_PV
  C1 : spsSeriesRLCBranchLib/Series RLC Branch  LConnTagsString=__new0  RConnTagsString=__new0  BranchType=C  Resistance=1.0  Inductance=1.0  SetiL0=off  InitialCurrent=0  Capacitance=0.00452266  Setx0=on  InitialVoltage=375/2  Measurements=None
  C2 : spsSeriesRLCBranchLib/Series RLC Branch  LConnTagsString=__new0  RConnTagsString=__new0  BranchType=C  Resistance=1.0  Inductance=1.0  SetiL0=off  InitialCurrent=0  Capacitance=0.00452266  Setx0=on  InitialVoltage=375/2  Measurements=None
  Cpv : spsThreePhaseSeriesRLCLoadLib/Three-Phase Series RLC Load  LConnTagsString=A|B|C  Configuration=Delta  NominalVoltage=195.1937  Vabc=[1e3 1e3 1e3]  Vabcp=[1e3 1e3 1e3]  NominalFrequency=50  UnbalancedPower=off  ActivePower=21.2  InductivePower=0  CapacitivePower=1060  Pabc=[10e3 9e3 11e3]  QLabc=[100 90 110]  QCabc=[100 90 110]  Pabcp=[10e3 9e3 11e3]  QLabcp=[100 90 110]  QCabcp=[100 90 110]  Measurements=None  LoadType=constant Z
  Inverter Control : Subsystem  mask(Inverter Control){Pnom=10600, Fnom=50, Vnom_prim=400, Vnom_sec=195.1937, Vnom_dc=375, Increment_MPPT=0.01, Limits_MPPT=[ 457 280 ], Vdc_ref_Init=375, Kp_VDCreg=2, Ki_VDCreg=400, Kp_Ireg=0.3, Ki_Ireg=20, RLff=[ 0.0039 0.21 ], Fc=1650, Ts_Control=6.06e-5, Ts_PWMgenerator=6.06e-6}
      mask prompts: Pnom "Power (VA)"; Fnom "Frequency (Hz)"; Vnom_prim "Primary voltage (Vrms LL)"; Vnom_sec "Secondary voltage (Vrms LL)"; Vnom_dc "DC voltage (V)"; Increment_MPPT "Output increment (V)"; Limits_MPPT "Output limits [ Upper  Lower ]"; Vdc_ref_Init "Output initial value (V)"; Kp_VDCreg "Proportional gain"; Ki_VDCreg "Integral gain"; Kp_Ireg "Proportional gain"; Ki_Ireg "Integral gain"; RLff "Feedforward Values [Rff Lff]"; Fc "Carrier frequency (Hz)"; Ts_Control "Control systems"; Ts_PWMgenerator "PWM generator"
      mask help:
      | The main components of the Inverter Control are:
      | 1. PLL & Measurements
      | 2. Maximum Power Point Tracker System (MPPT) using a Perturb & Observe algorithm
      | 3. DC Voltage Regulator
      | 4. Current Regulator
      | 5. PWM Modulator
      mask DialogControl Container4 Prompt: Nominal Values:
      mask DialogControl Container3 Prompt: MPPT Controller:
      mask DialogControl Container8 Prompt: Dc Voltage Regulator:
      mask DialogControl Container6 Prompt: Current Regulator:
      mask DialogControl Container9 Prompt: PWM Modulator:
      mask DialogControl SampleTimes Prompt: Sample Times:
  Irradiation(W/m^2) : spsStairGeneratorLib/Stair Generator  t=irradiation_time  e=irradiation_amplitude  Ts=0
  RL : spsThreePhaseSeriesRLCBranchLib/Three-Phase Series RLC Branch  LConnTagsString=A|B|C  RConnTagsString=A|B|C  BranchType=RL  Resistance=0.0053916  Inductance=0.001716197  Capacitance=inf  Measurements=None
  Rate Limiter : RateLimiter  RisingSlewLimit=6000  FallingSlewLimit=-6000  SampleTimeMode=inherited  InitialCondition=1000
  Saturation : Saturate  UpperLimit=55  LowerLimit=5
  Temp(degC) : spsStairGeneratorLib/Stair Generator  t=temperature_time  e=temperature_amplitude  Ts=0
  Tr1 : spsThreePhaseTransformerTwoWindingsLib/Three-Phase Transformer (Two Windings)  Winding1Connection=Yg  Winding2Connection=Delta (D1)  CoreType=Three single-phase transformers  SetSaturation=off  Hysteresis=off  DataFile='hysteresis'  SetInitialFlux=off  Measurements=None  UNITS=pu  NominalPower=[ 10600 50 ]  Winding1=[ 400 0.0012 0.03 ]  Winding2=[ 195.1937 0.0012 0.03 ]  Rm=200  Lm=200  L0=0.5  Saturation=[ 0,0 ; 0.0024,1.2 ; 1.0,1.52 ]  InitialFluxes=[ 0.8 , -0.8 , 0.7 ]  BreakLoop=off  DiscreteSolver=Trapezoidal iterative  DataType=off  TransfoNumber=0
  "Vdc " : spsVoltageMeasurementLib/Voltage Measurement  Tag=PoWeRsYsTeMmEaSuReMeNt  PhasorSimulation=off  OutputType=Magnitude  PSBequivalent=0
  Vdc 1 : spsVoltageMeasurementLib/Voltage Measurement  Tag=PoWeRsYsTeMmEaSuReMeNt  PhasorSimulation=off  OutputType=Magnitude  PSBequivalent=0
  A : PMIOPort  Side=Right
  B : PMIOPort  Port=2  Side=Right
  C : PMIOPort  Port=3  Side=Right
  tag scope: Irr=global, Temp_degC=global, Vab_VSC=global, Vdc_meas=global, meas_PV=global
  wires:
  Bus Selector/2 -> Inverter Control/5(I_PV)  "<I_PV>"
  Inverter Control/1(g) -> 3-Level IGBTs Bridge/1
  Rate Limiter/1 -> [Irr], 10.6kW/375V/28.5A/1
  Irradiation(W/m^2)/1 -> Rate Limiter/1
  [meas_PV] -> Bus Selector/1
  [Iabc_B1] -> Inverter Control/2(Iabc_prim)
  "Vdc "/1 -> [Vdc_meas]
  Vdc 1/1 -> [Vab_VSC]
  10.6kW/375V/28.5A/1 -> [meas_PV]
  [Vabc_B1] -> Inverter Control/1(Vabc_prim)
  [Vdc_meas] -> Inverter Control/3(Vdc_meas)
  Saturation/1 -> [Temp_degC], 10.6kW/375V/28.5A/2
  Temp(degC)/1 -> Saturation/1
  Bus Selector/1 -> Inverter Control/4(V_PV)  "<V_PV>"
  connections:
  3-Level IGBTs Bridge/RConn2 -- C1/RConn1 -- C2/LConn1
  "Vdc "/LConn1 -- 10.6kW/375V/28.5A/RConn1 -- 3-Level IGBTs Bridge/RConn1 -- C1/LConn1
  Cpv/LConn3 -- Tr1/RConn3 -- RL/RConn3
  Tr1/RConn1 -- Cpv/LConn1 -- RL/RConn1
  3-Level IGBTs Bridge/RConn3 -- 10.6kW/375V/28.5A/RConn2 -- "Vdc "/LConn2 -- C2/RConn1
  3-Level IGBTs Bridge/LConn2 -- RL/LConn2 -- Vdc 1/LConn2
  RL/RConn2 -- Tr1/RConn2 -- Cpv/LConn2
  3-Level IGBTs Bridge/LConn1 -- Vdc 1/LConn1 -- RL/LConn1
  B1/RConn1 -- A/RConn1
  B1/LConn2 -- Tr1/LConn2
  B1/LConn1 -- Tr1/LConn1
  RL/LConn3 -- 3-Level IGBTs Bridge/LConn3
  B1/LConn3 -- Tr1/LConn3
  B1/RConn2 -- B/RConn1
  B1/RConn3 -- C/RConn1

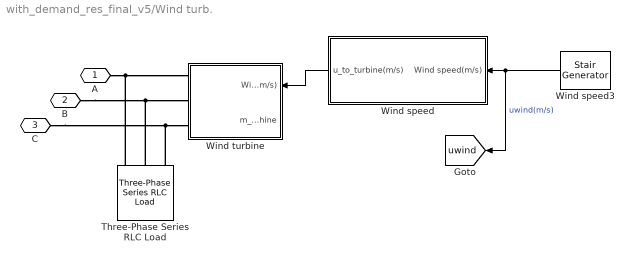
== system with_demand_res_final_v5/Wind turb. ==
  Three-Phase Series RLC Load : spsThreePhaseSeriesRLCLoadLib/Three-Phase Series RLC Load  LConnTagsString=A|B|C  Configuration=Y (grounded)  NominalVoltage=400  Vabc=[1e3 1e3 1e3]  Vabcp=[1e3 1e3 1e3]  NominalFrequency=50  UnbalancedPower=off  ActivePower=1e-6  InductivePower=0  CapacitivePower=18.6e3  Pabc=[10e3 9e3 11e3]  QLabc=[100 90 110]  QCabc=[100 90 110]  Pabcp=[10e3 9e3 11e3]  QLabcp=[100 90 110]  QCabcp=[100 90 110]  Measurements=None  LoadType=constant Z
  Wind speed : Subsystem
  Wind speed3 : spsStairGeneratorLib/Stair Generator  t=uwind_time  e=uwind_amplitude  Ts=0
  Wind turbine : Subsystem
      settings: PortSchema="{\"entries\":[{\"content\":{\"sides\":[{\"content\":{\"connectorIds\":[\"LConn1\",\"LConn2\",\"LConn3\"]},\"type\":\"ConnectorPlacement.EquallySpacedRectSide\",\"uuid\":\"08b69726-1df5-4ca6-8c10-95a87e57958a\"},{\"content\":{\"connectorIds\":[\"In1\",\"Out1\"],\"side\":\"RIGHT\"},\"type\":\"ConnectorPlacement.EquallySpacedRectSide\",\"uuid\":\"4b04fe79-4781-4367-afff-b10c5d568099\"},{\"content\":{\"side\":\"TOP\"},\"type\":\"ConnectorPlacement.EquallySpacedRectSide\",\"uuid\":\"2a53e08c-afc6-4d8a-b9a1-c6221c3edf36\"}]},\"type\":\"ConnectorPlacement.EquallySpacedConnector\",\"uuid\":\"1c063288-1d34-4ac9-8903-84a9f43e3a12\"}],\"packageUris\":[\"http://schema.mathworks.com/mf0/Connector/R2020b\"],\"version\":\"1.0\"}"
  A : PMIOPort  Side=Left
  B : PMIOPort  Port=2  Side=Left
  C : PMIOPort  Port=3  Side=Left
  tag scope: uwind=global
  wires:
  Wind speed/1(u_to_turbine(m/s)) -> Wind turbine/1("Wind (m/s) ")
  Wind speed3/1 -> [uwind], Wind speed/1(Wind speed(m/s))  "uwind(m/s)"
  connections:
  Three-Phase Series RLC Load/LConn2 -- B/RConn1 -- Wind turbine/LConn2
  Three-Phase Series RLC Load/LConn3 -- C/RConn1 -- Wind turbine/LConn3
  Three-Phase Series RLC Load/LConn1 -- A/RConn1 -- Wind turbine/LConn1

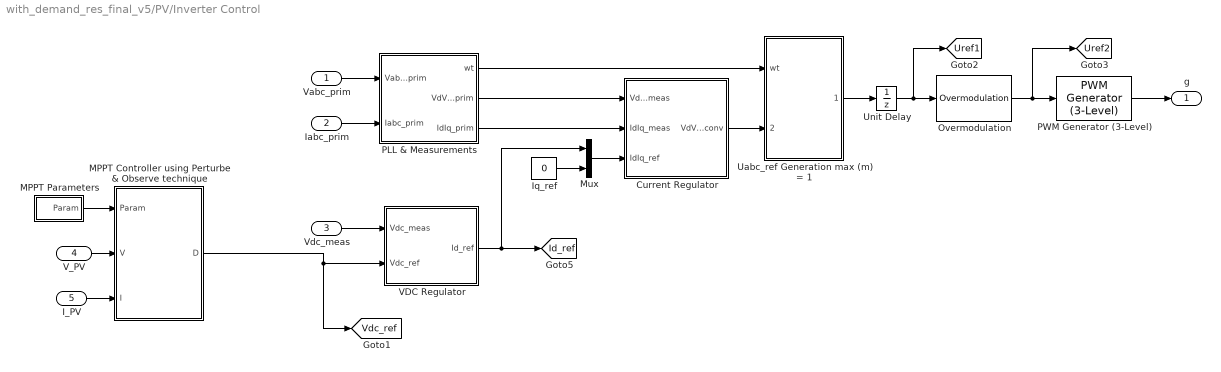
== system with_demand_res_final_v5/PV/Inverter Control ==
  Vabc_prim : Inport  PortDimensions=3
  Iabc_prim : Inport  Port=2  PortDimensions=3
  Vdc_meas : Inport  Port=3  PortDimensions=1
  V_PV : Inport  Port=4  PortDimensions=1
  I_PV : Inport  Port=5  PortDimensions=1
  Current Regulator : Subsystem
  Iq_ref : Constant  Value=0
  MPPT Parameters : Subsystem
  "MPPT Controller using Perturbe & Observe technique " : MATLAB Function  TreatAsAtomicUnit=on
  Mux : Mux  Inputs=2
  Overmodulation : spsOvermodulationLib/Overmodulation  OverModType=Flat top
      settings: LibrarySourceBlock=sps_lib/Power Electronics/Power Electronics Control/Overmodulation
  PLL & Measurements : Subsystem
  PWM Generator (3-Level) : spsPWMGenerator3LevelLib/PWM Generator (3-Level)  ModulatorType=Three-phase bridge (12 pulses)  ModulatorMode=Unsynchronized  nF=27  Fc=1650  ModulatingSignals=off  m=0.8  Freq=60  Phase=0  Ts=6.06e-6
      settings: LibrarySourceBlock=|
      | sps_lib/Power Electronics/Power Electronics Control/PWM Generator
      | (3-Level)
  Uabc_ref Generation max (m) = 1 : Subsystem
  Unit Delay : UnitDelay  SampleTime=6.06e-5  HasFrameUpgradeWarning=on
  VDC Regulator : Subsystem
  g : Outport  VectorParamsAs1DForOutWhenUnconnected=off
  tag scope: Id_ref=global, Uref1=global, Uref2=global, Vdc_ref=global
  wires:
  PLL & Measurements/1(wt) -> Uabc_ref Generation max (m) = 1/1(wt)
  Current Regulator/1(VdVq_conv) -> Uabc_ref Generation max (m) = 1/2(VdVq_conv)
  Iq_ref/1 -> Mux/2
  Mux/1 -> Current Regulator/3(IdIq_ref)
  PLL & Measurements/3(IdIq_prim) -> Current Regulator/2(IdIq_meas)
  PLL & Measurements/2(VdVq_prim) -> Current Regulator/1(VdVq_meas)
  Vabc_prim/1 -> PLL & Measurements/1(Vabc_prim)
  Iabc_prim/1 -> PLL & Measurements/2(Iabc_prim)
  PWM Generator (3-Level)/1 -> g/1
  Vdc_meas/1 -> VDC Regulator/1(Vdc_meas)
  VDC Regulator/1(Id_ref) -> [Id_ref], Mux/1
  V_PV/1 -> "MPPT Controller using Perturbe & Observe technique "/2(V)
  I_PV/1 -> "MPPT Controller using Perturbe & Observe technique "/3(I)
  MPPT Parameters/1(Param) -> "MPPT Controller using Perturbe & Observe technique "/1(Param)
  Overmodulation/1 -> [Uref2], PWM Generator (3-Level)/1
  Unit Delay/1 -> [Uref1], Overmodulation/1
  "MPPT Controller using Perturbe & Observe technique "/1(D) -> [Vdc_ref], VDC Regulator/2(Vdc_ref)
  Uabc_ref Generation max (m) = 1/1(Uabc_ref) -> Unit Delay/1

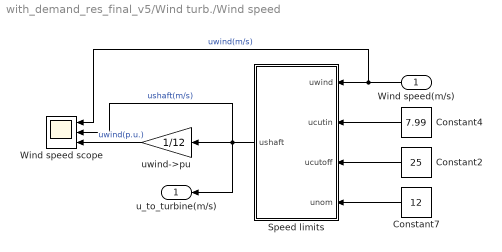
== system with_demand_res_final_v5/Wind turb./Wind speed ==
  Wind speed(m/s) : Inport
  Constant2 : Constant  Value=25
  Constant4 : Constant  Value=7.99
  Constant7 : Constant  Value=12
  Speed limits : MATLAB Function  TreatAsAtomicUnit=on
  Wind speed scope : Scope  NumInputPorts=3
  uwind->pu : Gain  Gain=1/12
  u_to_turbine(m/s) : Outport
  wires:
  Speed limits/1(ushaft) -> u_to_turbine(m/s)/1, uwind->pu/1, Wind speed scope/2  "ushaft(m/s)"
  Wind speed(m/s)/1 -> Wind speed scope/1, Speed limits/1(uwind)  "uwind(m/s)"
  Constant4/1 -> Speed limits/2(ucutin)
  uwind->pu/1 -> Wind speed scope/3  "uwind(p.u.)"
  Constant2/1 -> Speed limits/3(ucutoff)
  Constant7/1 -> Speed limits/4(unom)

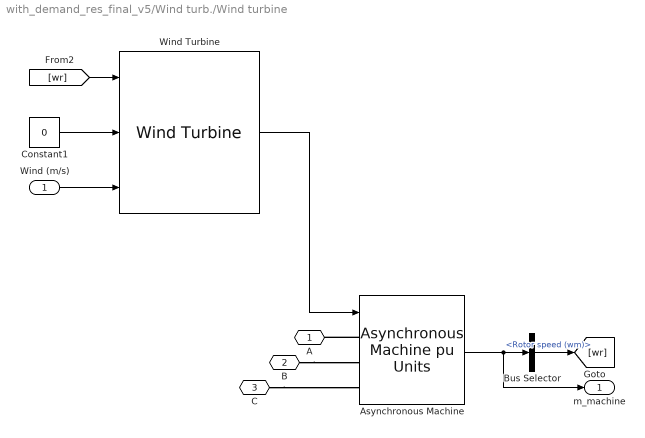
== system with_demand_res_final_v5/Wind turb./Wind turbine ==
  "Wind (m/s) " : Inport
  Asynchronous Machine : spsAsynchronousMachinepuUnitsLib/Asynchronous Machine pu Units  RotorType=Squirrel-cage  PresetModel=No  MechanicalLoad=Torque Tm  ShowDetailedParameters=on  ReferenceFrame=Rotor  Units=pu  MeasurementBus=off  NominalParameters=[ 27778 400 50 ]  VoltageRatio=1  Stator=[ 0.004843 0.1248]  Rotor=[ 0.007377 0.1791]  Cage1=[0.01909 0.0397]  Cage2=[0.01909 0.0397]  Lm=6.77  Mechanical=[ 5.04 0.001 3 ]  PolePairs=3  InitialConditions="[ -0.01,0,   0,0,0,   0,0,-0 ]"  SimulateSaturation=off  Saturation=[ 0 0 ; 0 0 ]  LoadFlowParameters=0  TsPowergui=0  TsBlock=-1  IterativeModel=Trapezoidal non iterative  IterativeDiscreteModel=Trapezoidal non iterative  Pmec=0
  Bus Selector : BusSelector  OutputSignals=Mechanical.Rotor speed (wm)
  Constant1 : Constant  Value=0
  Wind Turbine : spsWindTurbineLib/Wind Turbine  Pnom=25000  Pelec_base=27778  wind_base=12  P_wind_base=1  speed_nom=1  pitch_angle=0  c1_c6="[0.51763          116          0.4            5           21     0.006795]"  cp_nom=0.48  lambda_nom=8.1
  A : PMIOPort  Side=Left
  B : PMIOPort  Port=2  Side=Left
  C : PMIOPort  Port=3  Side=Left
  m_machine : Outport
  wires:
  [wr] -> Wind Turbine/1
  "Wind (m/s) "/1 -> Wind Turbine/3
  Asynchronous Machine/1 -> Bus Selector/1, m_machine/1
  Wind Turbine/1 -> Asynchronous Machine/1
  Bus Selector/1 -> [wr]  "<Rotor speed (wm)>"
  Constant1/1 -> Wind Turbine/2
  connections:
  Asynchronous Machine/LConn1 -- A/RConn1
  B/RConn1 -- Asynchronous Machine/LConn2
  C/RConn1 -- Asynchronous Machine/LConn3

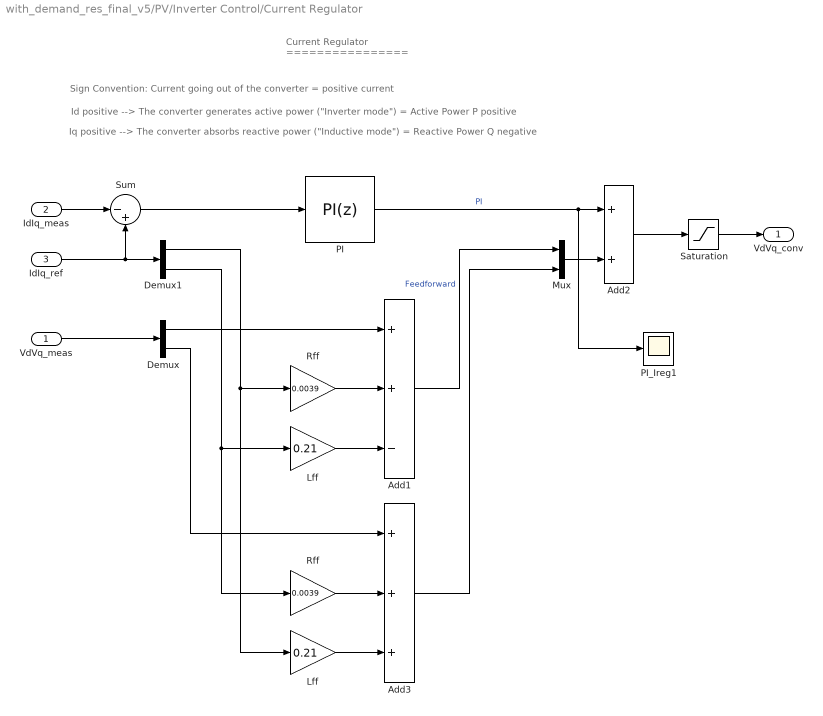
== system with_demand_res_final_v5/PV/Inverter Control/Current Regulator ==
  note: Current Regulator
      | ================
  note: Sign Convention: Current going out of the converter = positive current
  note: Iq positive --> The converter absorbs reactive power ("Inductive mode") = Reactive Power Q negative
  note: Id positive --> The converter generates active power ("Inverter mode") = Active Power P positive
  VdVq_meas : Inport  PortDimensions=2
  IdIq_meas : Inport  Port=2  PortDimensions=2
  IdIq_ref : Inport  Port=3  PortDimensions=2
  Add1 : Sum  Inputs=++-
  Add2 : Sum
  Add3 : Sum  Inputs=+++
  Demux : Demux  Outputs=2
  Demux1 : Demux  Outputs=2
  Lff : Gain  Gain=0.21  SaturateOnIntegerOverflow=on  OutDataTypeStr=Inherit: Same as input  ParamDataTypeStr=Inherit: Same as input
  "Lff  " : Gain  Gain=0.21  SaturateOnIntegerOverflow=on  OutDataTypeStr=Inherit: Same as input  ParamDataTypeStr=Inherit: Same as input
  Mux : Mux  Inputs=2
  PI : slpidlib/PID Controller  Controller=PI  Form=Parallel  TimeDomain=Discrete-time  UseExternalTs=off  SampleTime=Ts_Control  IntegratorMethod=Forward Euler  FilterMethod=Forward Euler  ControllerParametersSource=internal  P=0.3  I=20  UseKiTs=off  D=0  UseExternalDerivativeSource=off  N=100  UseFilter=on  TunerSelectOption=Transfer Function Based (PID Tuner App)  InitialConditionSource=internal  InitialConditionForIntegrator=0  InitialConditionForFilter=0  DifferentiatorICPrevScaledInput=0  ExternalReset=none  TrackingMode=off  Kt=1  LimitOutput=on  SatLimitsSource=internal  UpperSaturationLimit=1.5  LowerSaturationLimit=-1.5  LinearizeAsGain=off  AntiWindupMode=none  Kb=1  LimitIntegrator=off  UpperIntegratorSaturationLimit=inf  LowerIntegratorSaturationLimit=-inf  POutMin=[]  POutMax=[]  IOutMin=[]  IOutMax=[]  DOutMin=[]  DOutMax=[]  NOutMin=[]  NOutMax=[]  SumOutMin=[]  SumOutMax=[]  SaturationOutMin=[]  SaturationOutMax=[]  PParamMin=[]  PParamMax=[]  IParamMin=[]  IParamMax=[]  DParamMin=[]  DParamMax=[]  NParamMin=[]  NParamMax=[]  KbParamMin=[]  KbParamMax=[]  KtParamMin=[]  KtParamMax=[]  KbOutMin=[]  KbOutMax=[]  KtOutMin=[]  KtOutMax=[]  IntegratorOutMin=[]  IntegratorOutMax=[]  FilterOutMin=[]  FilterOutMax=[]  SumI1OutMin=[]  SumI1OutMax=[]  SumI2OutMin=[]  SumI2OutMax=[]  SumI3OutMin=[]  SumI3OutMax=[]  SumI4OutMin=[]  SumI4OutMax=[]  SumDOutMin=[]  SumDOutMax=[]  DifferentiatorOutMin=[]  DifferentiatorOutMax=[]  FilterDiffOutCoefMin=[]  FilterDiffOutCoefMax=[]  ReciprocalOutMin=[]  ReciprocalOutMax=[]  SumDenOutMin=[]  SumDenOutMax=[]  SumNumOutMin=[]  SumNumOutMax=[]  DivideOutMin=[]  DivideOutMax=[]  UdiffTsProdOutMin=[]  UdiffTsProdOutMax=[]  NTsProdOutMin=[]  NTsProdOutMax=[]  UintegralTsProdOutMin=[]  UintegralTsProdOutMax=[]  UngainTsProdOutMin=[]  UngainTsProdOutMax=[]  ClampingZeroOutDataTypeStr=Inherit: Inherit via back propagation  ClampingZeroOutMin=[]  ClampingZeroOutMax=[]  FilterDenConstantOutDataTypeStr=Inherit: Inherit via back propagation  FilterDenConstantOutMin=[]  FilterDenConstantOutMax=[]  PCopyOutDataTypeStr=Inherit: Inherit via back propagation  PCopyOutMin=[]  PCopyOutMax=[]  NCopyOutDataTypeStr=Inherit: Inherit via back propagation  NCopyOutMin=[]  NCopyOutMax=[]  IntegratorContinuousStateAttributes=''  IntegratorStateMustResolveToSignalObject=off  IntegratorRTWStateStorageClass=Auto  FilterContinuousStateAttributes=''  FilterStateMustResolveToSignalObject=off  FilterRTWStateStorageClass=Auto  ParallelPVariant=InternalParameters  IdealPVariant=Disabled  IVariant=InternalParameters  DVariant=Disabled  IntegratorVariant=Discrete  SatVariant=Enabled  AWVariant=Passthrough  PCopyVariant=Disabled  TRVariant=Disabled  FdbkBlocksVariant=Forward  IdealPFdbkVariant=Disabled  SatFdbkVariant=Disabled  DerivativeFilterVariant=Disabled  NVariant=Disabled  NCopyVariant=Disabled_SignalSpec  FilterICVariant=Disabled  IntegratorICVariant=InternalICs  ExternalResetVariant=Disabled  TRSumVariant=Passthrough  SumFdbkVariant=Disabled  SumVariant=Sum_PI  TsampFilterVariant=InternalTs  TsampNgainVariant=Passthrough  TsampIntegralVariant=Disabled_SignalSpec  ExternalSaturationOutDataTypeStr=Inherit: Same as second input  DerivativeSourceVariant=Disabled
  PI_Ireg1 : Scope
  Rff : Gain  Gain=0.0039  SaturateOnIntegerOverflow=on  OutDataTypeStr=Inherit: Same as input  ParamDataTypeStr=Inherit: Same as input
  "Rff " : Gain  Gain=0.0039  SaturateOnIntegerOverflow=on  OutDataTypeStr=Inherit: Same as input  ParamDataTypeStr=Inherit: Same as input
  Saturation : Saturate  UpperLimit=1.5  LowerLimit=-1.5
  Sum : Sum  Inputs=|-+
  VdVq_conv : Outport  VectorParamsAs1DForOutWhenUnconnected=off
  wires:
  Mux/1 -> Add2/2
  PI/1 -> PI_Ireg1/1, Add2/1  "PI"
  Sum/1 -> PI/1
  IdIq_ref/1 -> Sum/2, Demux1/1
  IdIq_meas/1 -> Sum/1
  Add2/1 -> Saturation/1
  Saturation/1 -> VdVq_conv/1
  VdVq_meas/1 -> Demux/1
  Demux/1 -> Add1/1
  "Rff "/1 -> Add1/2
  Demux1/1 -> "Rff "/1, Lff/1
  "Lff  "/1 -> Add1/3
  Demux1/2 -> "Lff  "/1, Rff/1
  Rff/1 -> Add3/2
  Lff/1 -> Add3/3
  Add1/1 -> Mux/1  "Feedforward"
  Demux/2 -> Add3/1
  Add3/1 -> Mux/2

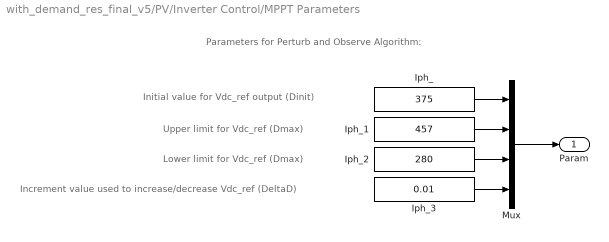
== system with_demand_res_final_v5/PV/Inverter Control/MPPT Parameters ==
  note: Parameters for Perturb and Observe Algorithm:
  note: Lower limit for Vdc_ref (Dmax)
  note: Initial value for Vdc_ref output (Dinit)
  note: Increment value used to increase/decrease Vdc_ref (DeltaD)
  note: Upper limit for Vdc_ref (Dmax)
  Iph_ : Constant  Value=375
  Iph_1 : Constant  Value=457
  Iph_2 : Constant  Value=280
  Iph_3 : Constant  Value=0.01
  Mux : Mux
  Param : Outport  VectorParamsAs1DForOutWhenUnconnected=off
  wires:
  Mux/1 -> Param/1
  Iph_3/1 -> Mux/4
  Iph_2/1 -> Mux/3
  Iph_1/1 -> Mux/2
  Iph_/1 -> Mux/1

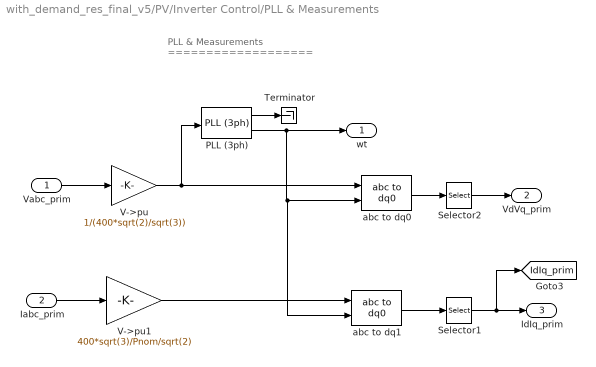
== system with_demand_res_final_v5/PV/Inverter Control/PLL & Measurements ==
  note: PLL & Measurements
      | ===================
  Vabc_prim : Inport
  Iabc_prim : Inport  Port=2
  PLL (3ph) : spsPLL3phLib/PLL (3ph)  Fmin=45  Par_Init="[-0.57  50]"  ParK=[180, 3200, 1]  TcD=1e-4  MaxRateChangeFreq=12  FilterCutOffFreq=25  Ts=6.06e-5  AGC=on
  Selector1 : Selector  InputPortWidth=3  IndexOptions=Index vector (dialog)  Indices=[1 2]  OutputSizes=1
  Selector2 : Selector  InputPortWidth=3  IndexOptions=Index vector (dialog)  Indices=[1 2]  OutputSizes=1
  Terminator : Terminator
  V->pu : Gain  Gain=1/(400*sqrt(2)/sqrt(3))  SaturateOnIntegerOverflow=on  OutDataTypeStr=Inherit: Same as input  ParamDataTypeStr=Inherit: Same as input
  V->pu1 : Gain  Gain=400*sqrt(3)/Pnom/sqrt(2)  SaturateOnIntegerOverflow=on  OutDataTypeStr=Inherit: Same as input  ParamDataTypeStr=Inherit: Same as input
  abc to dq0 : spsabctodq0Lib/abc to dq0  Alignment=90 degrees behind phase A axis
  abc to dq1 : spsabctodq0Lib/abc to dq0  Alignment=90 degrees behind phase A axis
  wt : Outport  VectorParamsAs1DForOutWhenUnconnected=off
  VdVq_prim : Outport  Port=2  VectorParamsAs1DForOutWhenUnconnected=off
  IdIq_prim : Outport  Port=3  VectorParamsAs1DForOutWhenUnconnected=off
  tag scope: IdIq_prim=global
  wires:
  V->pu1/1 -> abc to dq1/1
  V->pu/1 -> PLL (3ph)/1, abc to dq0/1
  abc to dq1/1 -> Selector1/1
  Vabc_prim/1 -> V->pu/1
  Iabc_prim/1 -> V->pu1/1
  abc to dq0/1 -> Selector2/1
  Selector2/1 -> VdVq_prim/1
  Selector1/1 -> [IdIq_prim], IdIq_prim/1
  PLL (3ph)/2 -> wt/1, abc to dq1/2, abc to dq0/2
  PLL (3ph)/1 -> Terminator/1

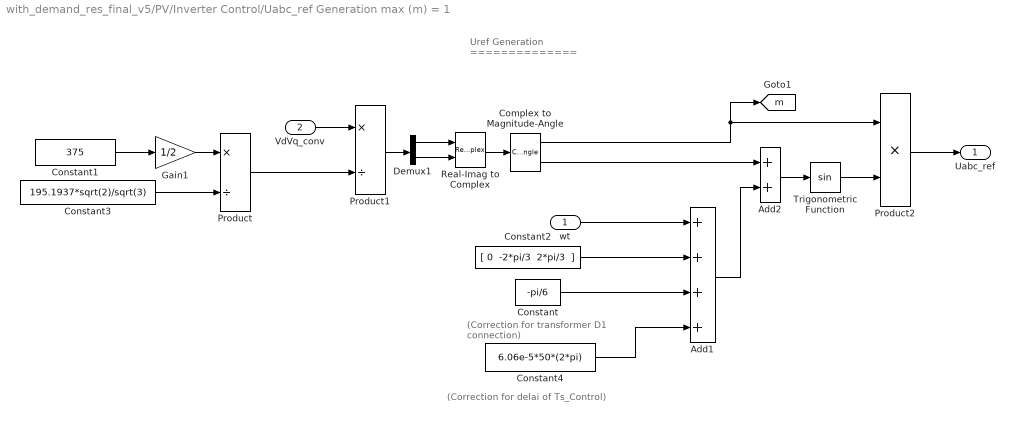
== system with_demand_res_final_v5/PV/Inverter Control/Uabc_ref Generation max (m) = 1 ==
  note: (Correction for transformer
      |  D1 connection)
  note: (Correction for delai of Ts_Control)
  note: Uref Generation
      | ==============
  wt : Inport
  VdVq_conv : Inport  Port=2
  Add1 : Sum  Inputs=++++
  Add2 : Sum
  Complex to Magnitude-Angle : ComplexToMagnitudeAngle
  Constant : Constant  Value=-pi/6
  Constant1 : Constant  Value=375
  Constant2 : Constant  Value="[ 0  -2*pi/3  2*pi/3  ]"
  Constant3 : Constant  Value=195.1937*sqrt(2)/sqrt(3)
  Constant4 : Constant  Value=6.06e-5*50*(2*pi)
  Demux1 : Demux  Outputs=2
  Gain1 : Gain  Gain=1/2
  Product : Product  Inputs=*/  RndMeth=Zero
  Product1 : Product  Inputs=*/  RndMeth=Zero
  Product2 : Product  Inputs=**  RndMeth=Zero
  Real-Imag to Complex : RealImagToComplex
  Trigonometric Function : Trigonometry
  Uabc_ref : Outport  VectorParamsAs1DForOutWhenUnconnected=off
  tag scope: m=global
  wires:
  Constant1/1 -> Gain1/1
  VdVq_conv/1 -> Product1/1
  Product1/1 -> Demux1/1
  Gain1/1 -> Product/1
  Real-Imag to Complex/1 -> Complex to Magnitude-Angle/1
  Demux1/1 -> Real-Imag to Complex/1
  Demux1/2 -> Real-Imag to Complex/2
  Constant2/1 -> Add1/2
  Constant/1 -> Add1/3
  Constant3/1 -> Product/2
  Product/1 -> Product1/2
  Complex to Magnitude-Angle/2 -> Add2/1
  Add1/1 -> Add2/2
  Add2/1 -> Trigonometric Function/1
  Complex to Magnitude-Angle/1 -> [m], Product2/1
  Trigonometric Function/1 -> Product2/2
  Product2/1 -> Uabc_ref/1
  wt/1 -> Add1/1
  Constant4/1 -> Add1/4
